simulink model "SIL_Arduino"  (R2022b)
settings: Solver=ode3  StartTime=0.0  StopTime=10.0  FixedStep=0.01  RelTol=1e-3
values from neighbouring files (symbols this model uses):
  Acceleration_Max = 3.2    [Matlab_WorkSpace.mat]
  Distance_initial = 8    [Matlab_WorkSpace.mat]
  Frein_Max = -9    [Matlab_WorkSpace.mat]
  glissement = 0.22    [Matlab_WorkSpace.mat]
  r = 0.3    [Matlab_WorkSpace.mat]
  vehicule_half_length = 2.5    [Matlab_WorkSpace.mat]
libraries: sim3dautolib x2, sim3dprobsensorlib x1, sim3dlib x1, pil_lib x1, slpidlib x1
settings Model: Creator=Yoamiri  LastModifiedBy=Yoamiri
settings OptimizationCC: DefaultParameterBehavior=Inlined  EnhancedBackFolding=on  PassReuseOutputArgsAs=Individual arguments  ZeroExternalMemoryAtStartup=off  ZeroInternalMemoryAtStartup=off  OptimizeBlockOrder=speed  DifferentSizesBufferReuse=on  OptimizationCustomize=off  EfficientTunableParamExpr=on
settings DebuggingCC: ParameterPrecisionLossMsg=none  ParameterTunabilityLossMsg=error
settings HardwareCC: ProdBitPerPointer=32  ProdBitPerSizeT=32  ProdBitPerPtrDiffT=32  ProdLargestAtomicFloat=None  ProdWordSize=32  ProdHWDeviceType=Atmel->AVR (32-bit)
settings SFSimCC: MATLABDynamicMemAlloc=off
settings RTWCC: Description=Embedded Coder  SystemTargetFile=ert.tlc  TemplateMakefile=ert_default_tmf  CreateSILPILBlock=SIL
settings CodeAppCC: ForceParamTrailComments=on  IgnoreCustomStorageClasses=off  OperatorAnnotations=on  SimulinkDataObjDesc=on  SFDataObjDesc=on  InsertBlockDesc=on
settings ERTTargetCC: TargetLangStandard=C99 (ISO)  GenerateSampleERTMain=on  SupportContinuousTime=on  SupportVariableSizeSignals=on  InlinedParameterPlacement=NonHierarchical  ERTCustomFileTemplate=example_file_process.tlc

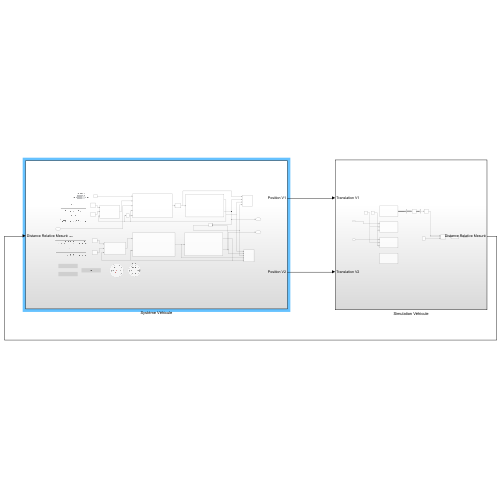
[thumbnail: Simulink's stored preview of the top-level diagram]
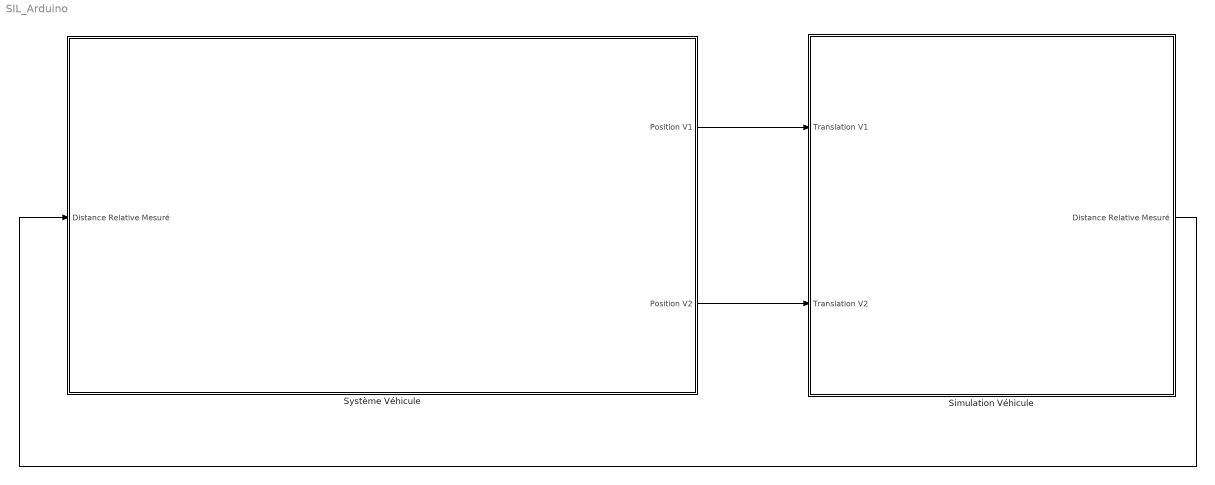
== system SIL_Arduino ==
  Simulation Véhicule : Subsystem
  Système Véhicule : Subsystem
  wires:
  Simulation Véhicule/1(Distance Relative Mesuré) -> Système Véhicule/1(Distance Relative Mesuré)
  Système Véhicule/2(Position V2) -> Simulation Véhicule/2(Translation V2)
  Système Véhicule/1(Position V1) -> Simulation Véhicule/1(Translation V1)

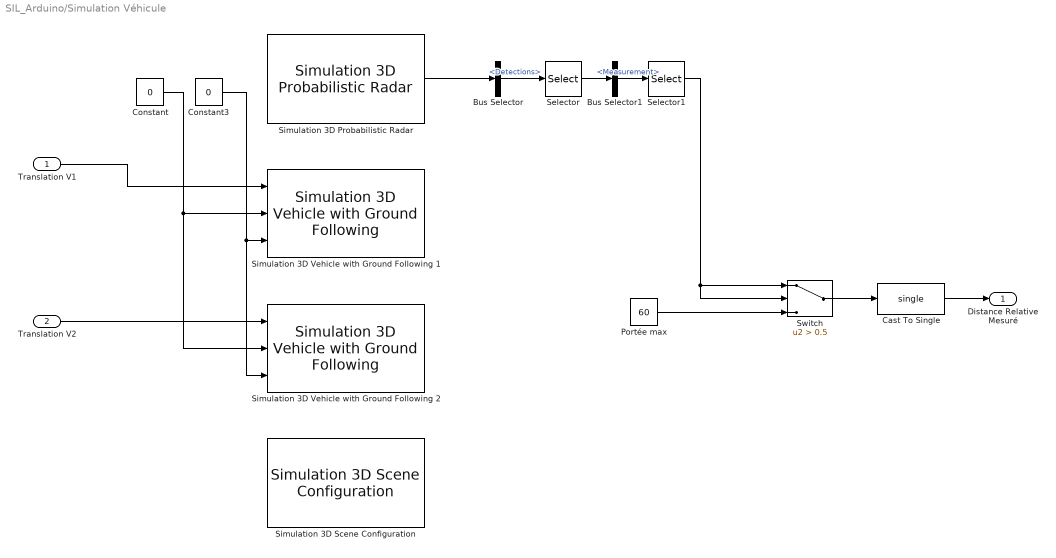
== system SIL_Arduino/Simulation Véhicule ==
  Translation V1 : Inport
  Translation V2 : Inport  Port=2
  Bus Selector : BusSelector  OutputSignals=Detections
  Bus Selector1 : BusSelector  OutputSignals=Measurement
  Cast To Single : DataTypeConversion  OutDataTypeStr=single  SaturateOnIntegerOverflow=off  RndMeth=Floor
  Constant : Constant  Value=0
  Constant3 : Constant  Value=0
  Portée max : Constant  Value=60
  Selector : Selector  InputPortWidth=50  IndexOptions=Index vector (dialog)  Indices=[1]  OutputSizes=1
  Selector1 : Selector  InputPortWidth=6  IndexOptions=Index vector (dialog)  Indices=[1]  OutputSizes=1
  Simulation 3D Probabilistic Radar : sim3dprobsensorlib/Simulation 3D Probabilistic Radar  Priority=1  sensorTag=Sim3dSensor2  sensorId=2  sensorName=Sim3dSensor2  vehTagList={'Scene Origin';'SimulinkVehicle1';'SimulinkVehicle2'}  vehTag=SimulinkVehicle1  mountLoc=Origin  offsetFlag=off  tmountOffset=[2.42, 0, 0.6]  rmountOffset=[0, 0, 0]  AzimuthResolution=4  ElevationResolution=10  RangeResolution=2.5  RangeRateResolution=0.5  AzimuthBiasFraction=0.1  ElevationBiasFraction=0.1  RangeBiasFraction=0.05  RangeRateBiasFraction=0.05  FieldOfView=[ 50, 10 ]  DetectionRange=[ 0.5, 200 ]  RangeRateLimits=[ -100, 100 ]  DetectionProbability=0.95  FalseAlarmRate=1e-6  ReferenceRange=180  ReferenceRCS=-10  HasElevation=on  HasRangeRate=on  HasNoise=on  HasFalseAlarms=on  InitialSeedSource=Repeatable  InitialSeed=0  MaxNumDetections=50  DetectionCoordinates=Ego Cartesian  SpecifyOutputBusName=off  BusName=BusSimulation3DRadarTruthSensor  SampleTime=-1  mountPoint=[0 0 0]  mountOrientation=[0 0 0]  aMode=3  ID=2
      settings: LibrarySourceBlock=drivingsim3d/Simulation 3D Probabilistic Radar
  Simulation 3D Scene Configuration : sim3dlib/Simulation 3D Scene Configuration  Priority=0  ProjectFormat=Default Scenes  SceneDesc=Straight road  ProjectName=C:\Program Files\MATLAB\R2022b\toolbox\shared\sim3d_projects\automotive_project\UE4\WindowsNoEditor\VehicleSimulation.exe  ScenePath=/Game/Maps/HwStrght  EnableOpenDRIVE=off  vehTagList={'Scene Origin';'SimulinkVehicle1';'SimulinkVehicle2'}  vehTag=SimulinkVehicle1  OpVisEn=off  Ts=1/20  EnableWindow=on  EnableRemoteAccess=off  EnableWeather=off  SunAltitude=40.0  SunAzimuth=90  clouds=10  wind=1  fog=0  rain=0  EnableGeospatial=off  OriginHeight=200  OriginLatitude=40.744652  OriginLongitude=-73.988864  MapStyle=Aerial  AdditionalAssetIDs=[]  UseAdvancedSunSky=off  SolarTime=11  TimeZone=-5  Day=21  Month=9  Year=2022  UseDaylightSavingTime=on  DSTStartDay=10  DSTStartMonth=3  DSTEndDay=3  DSTEndMonth=11  DSTSwitchHour=2  sensorTag=MainCamera2  sensorId=2  sensorName=MainCamera2  mountLoc=Origin  offsetFlag=off  tmountOffset=[0, 0, 0]  rmountOffset=[0, 0, 0]  HorizontalResolution=1280  VerticalResolution=720  HorizontalFOV=60  mountPoint=[0 0 0]  mountOrientation=[0 0 0]  aMode=3  ID=2  GeoTrigger=Inactive
      settings: LibrarySourceBlock=drivingsim3d/Simulation 3D Scene Configuration
  Simulation 3D Vehicle with Ground Following 1 : sim3dautolib/Simulation 3D Vehicle with Ground Following  Priority=-1  PassVehMesh=Sedan  MeshPath=/MathWorksAutomotiveContent/Vehicles/Muscle/Meshes/SK_MuscleCar.SK_MuscleCar  TrackWidth=1.9  WheelBase=3  WheelRadius=0.35  VehColor=Blue  InitialPos=[0, 0, 0]  InitialRot=[0, 0, 0]  ActorName=SimulinkVehicle3  SampleTime=-1  ActorType=SimulinkVehicle  ID=3  aMode=3  ActorTag=SimulinkVehicle3  CoordinateScheme=ISO  VehLightsControl=off  HeadlightColor=[ 1, 1, 1 ]  HighBeamIntensity=100000  LowBeamIntensity=60000  HighBeamConeAngle=70  LowBeamConeAngle=70  LeftHeadlightOrientation=[ 0, 0 ]  RightHeadlightOrientation=[ 0, 0 ]  BrakelightIntensity=500  ReverselightIntensity=500  SignallightIntensity=500  SignallightPeriod=1  SignalPulseWidth=50  TransformOutportEnabled=off
      settings: LibrarySourceBlock=drivingsim3d/Simulation 3D Vehicle with Ground Following
  Simulation 3D Vehicle with Ground Following 2 : sim3dautolib/Simulation 3D Vehicle with Ground Following  Priority=-1  PassVehMesh=Sedan  MeshPath=/MathWorksAutomotiveContent/Vehicles/Muscle/Meshes/SK_MuscleCar.SK_MuscleCar  TrackWidth=1.9  WheelBase=3  WheelRadius=0.35  VehColor=White  InitialPos=[0, 0, 0]  InitialRot=[0, 0, 0]  ActorName=SimulinkVehicle4  SampleTime=-1  ActorType=SimulinkVehicle  ID=4  aMode=3  ActorTag=SimulinkVehicle4  CoordinateScheme=ISO  VehLightsControl=off  HeadlightColor=[ 1, 1, 1 ]  HighBeamIntensity=100000  LowBeamIntensity=60000  HighBeamConeAngle=70  LowBeamConeAngle=70  LeftHeadlightOrientation=[ 0, 0 ]  RightHeadlightOrientation=[ 0, 0 ]  BrakelightIntensity=500  ReverselightIntensity=500  SignallightIntensity=500  SignallightPeriod=1  SignalPulseWidth=50  TransformOutportEnabled=off
      settings: LibrarySourceBlock=drivingsim3d/Simulation 3D Vehicle with Ground Following
  Switch : Switch  Criteria=u2 > Threshold  Threshold=0.5  SaturateOnIntegerOverflow=off  InputSameDT=off
  Distance Relative Mesuré : Outport
  wires:
  Constant/1 -> Simulation 3D Vehicle with Ground Following 1/2, Simulation 3D Vehicle with Ground Following 2/2
  Constant3/1 -> Simulation 3D Vehicle with Ground Following 2/3, Simulation 3D Vehicle with Ground Following 1/3
  Simulation 3D Probabilistic Radar/1 -> Bus Selector/1
  Bus Selector/1 -> Selector/1  "<Detections>"
  Selector/1 -> Bus Selector1/1
  Bus Selector1/1 -> Selector1/1  "<Measurement>"
  Translation V2/1 -> Simulation 3D Vehicle with Ground Following 2/1
  Translation V1/1 -> Simulation 3D Vehicle with Ground Following 1/1
  Switch/1 -> Cast To Single/1
  Selector1/1 -> Switch/1, Switch/2
  Portée max/1 -> Switch/3
  Cast To Single/1 -> Distance Relative Mesuré/1

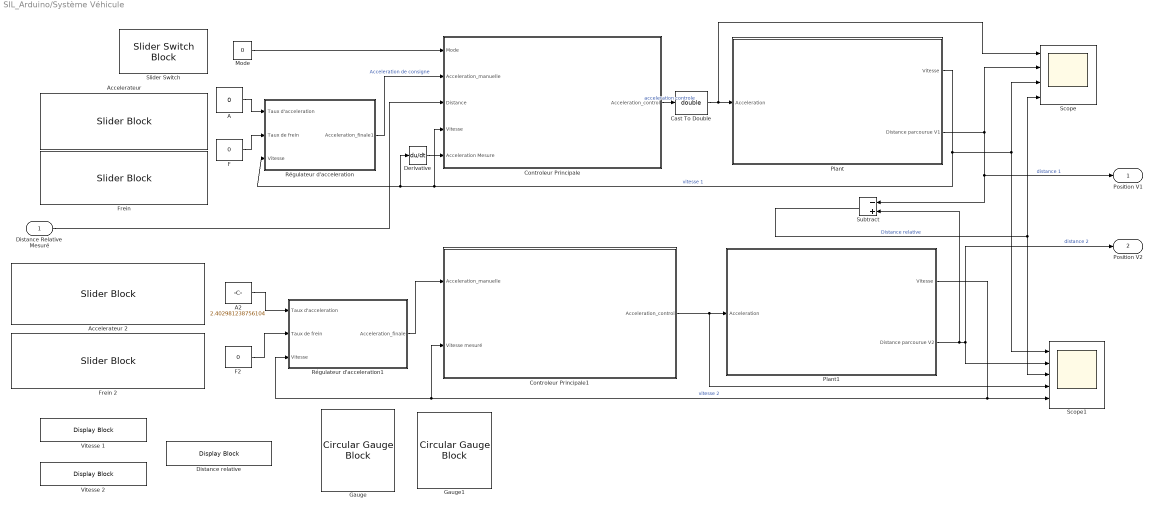
== system SIL_Arduino/Système Véhicule ==
  Distance Relative Mesuré : Inport
  A : Constant  Value=0
  A2 : Constant  Value=2.402981238756104
  Accelerateur : SliderBlock
  Accelerateur 2 : SliderBlock  TickInterval=10
  Cast To Double : DataTypeConversion  OutDataTypeStr=double  SaturateOnIntegerOverflow=off  RndMeth=Floor
  Controleur Principale : Subsystem  DialogController=pil_create_dialog  LoadFcn=|
      | try
      |    if ~strcmp(rtw.pil.getPILVersion, '9.13 (R2022b)_15')
      |       set_param(gcb, 'DialogController', '');
      |       set_param(gcb, 'DialogControllerArgs', '');
      |    end
      | catch e
      |       set_param(gcb, 'DialogController', '');
      |       set_param(gcb, 'DialogControllerArgs', '');
      | end
      mask help: PIL:pil:XILBlockMaskDesc
      mask Display: disp('SIL');
  Controleur Principale1 : Subsystem
  Derivative : Derivative
  Distance relative : DisplayBlock  LabelPosition=Hide  Transparency=1
  F : Constant  Value=0
  F2 : Constant  Value=0
  Frein : SliderBlock
  Frein 2 : SliderBlock  TickInterval=10
  Gauge : CircularGaugeBlock
  Gauge1 : CircularGaugeBlock
  Mode : Constant  Value=0  OutDataTypeStr=boolean
  Plant : Subsystem
  Plant1 : Subsystem
  Régulateur d'acceleration : Subsystem
  Régulateur d'acceleration1 : Subsystem
  Scope : Scope  NumInputPorts=4
  Scope1 : Scope  NumInputPorts=5
  Slider Switch : SliderSwitchBlock
      settings: Values={{'Off', 'On'}, [1 0]}
  Subtract : Sum  Inputs=-+
  Vitesse 1 : DisplayBlock  LabelPosition=Hide  Transparency=1
  Vitesse 2 : DisplayBlock  LabelPosition=Hide  Transparency=1
  Position V1 : Outport
  Position V2 : Outport  Port=2
  wires:
  Controleur Principale1/1(Acceleration_control) -> Plant1/1(Acceleration), Scope1/4
  A2/1 -> Régulateur d'acceleration1/1(Taux d'acceleration)
  Régulateur d'acceleration1/1(Acceleration_finale) -> Controleur Principale1/1(Acceleration_manuelle)
  Régulateur d'acceleration/1(Acceleration_finale1) -> Controleur Principale/2(Acceleration_manuelle)  "Acceleration de consigne"
  Controleur Principale/1(Acceleration_control) -> Cast To Double/1  "acceleration controle"
  F2/1 -> Régulateur d'acceleration1/2(Taux de frein)
  Plant/1(Vitesse) -> Scope/3, Scope1/1, Controleur Principale/4(Vitesse), Derivative/1, Régulateur d'acceleration/3(Vitesse)  "vitesse 1"
  Mode/1 -> Controleur Principale/1(Mode)
  Subtract/1 -> Scope/4, Scope1/3  "Distance relative"
  Plant1/1(Vitesse) -> Régulateur d'acceleration1/3(Vitesse), Controleur Principale1/2(Vitesse mesuré), Scope1/5  "vitesse 2"
  Plant/2(Distance parcourue V1) -> Scope/2, Position V1/1, Subtract/1  "distance 1"
  Plant1/2(Distance parcourue V2) -> Scope1/2, Position V2/1, Subtract/2  "distance 2"
  A/1 -> Régulateur d'acceleration/1(Taux d'acceleration)
  F/1 -> Régulateur d'acceleration/2(Taux de frein)
  Distance Relative Mesuré/1 -> Controleur Principale/3(Distance)
  Cast To Double/1 -> Scope/1, Plant/1(Acceleration)
  Derivative/1 -> Controleur Principale/5(Acceleration Mesure)

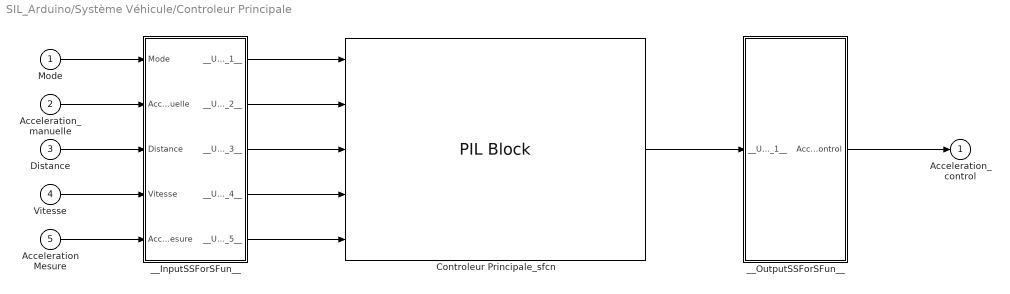
== system SIL_Arduino/Système Véhicule/Controleur Principale ==
  Mode : Inport
  Acceleration_manuelle : Inport  Port=2
  Distance : Inport  Port=3
  Vitesse : Inport  Port=4
  Acceleration Mesure : Inport  Port=5
  Controleur Principale_sfcn : pil_lib/PIL Block  SimulationMode=SIL  IsTopModelPIL=off  CodeDir=Controleur_ert_rtw  AnchorDir=C:\Users\Yoamiri\Desktop\Projet-Controle d'espacement en file de vehicules\MIL-Principale Modèle  ConfigName=Software-in-the-Loop (SIL)  XrelIsTopModelCode=on  XrelIsReusable=off  XrelDWorkNames={}  XrelDWorkTypes={}  XrelModelArgVals={}  XrelOrderedParamNames={}
  __InputSSForSFun__ : Subsystem
  __OutputSSForSFun__ : Subsystem
  Acceleration_control : Outport
  wires:
  Mode/1 -> __InputSSForSFun__/1(Mode)
  Acceleration_manuelle/1 -> __InputSSForSFun__/2(Acceleration_manuelle)
  Distance/1 -> __InputSSForSFun__/3(Distance)
  Vitesse/1 -> __InputSSForSFun__/4(Vitesse)
  Acceleration Mesure/1 -> __InputSSForSFun__/5(Acceleration Mesure)
  __InputSSForSFun__/1(__UniqueOutportName__1__) -> Controleur Principale_sfcn/1
  __InputSSForSFun__/2(__UniqueOutportName__2__) -> Controleur Principale_sfcn/2
  __InputSSForSFun__/3(__UniqueOutportName__3__) -> Controleur Principale_sfcn/3
  __InputSSForSFun__/4(__UniqueOutportName__4__) -> Controleur Principale_sfcn/4
  __InputSSForSFun__/5(__UniqueOutportName__5__) -> Controleur Principale_sfcn/5
  Controleur Principale_sfcn/1 -> __OutputSSForSFun__/1(__UniqueInportName__1__)
  __OutputSSForSFun__/1(Acceleration_control) -> Acceleration_control/1

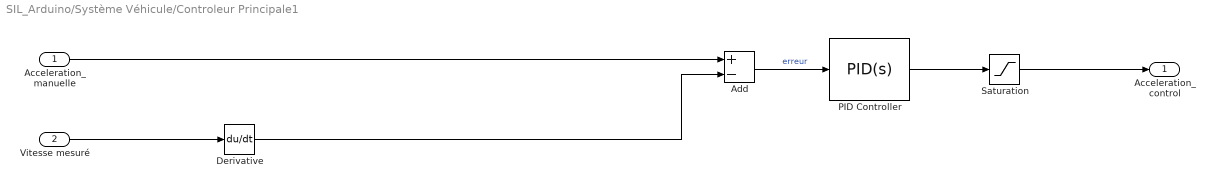
== system SIL_Arduino/Système Véhicule/Controleur Principale1 ==
  Acceleration_manuelle : Inport
  Vitesse mesuré : Inport  Port=2
  Add : Sum  Inputs=+-
  Derivative : Derivative
  PID Controller : slpidlib/PID Controller  Controller=PID  Form=Parallel  TimeDomain=Continuous-time  UseExternalTs=off  SampleTime=-1  IntegratorMethod=Forward Euler  FilterMethod=Forward Euler  ControllerParametersSource=internal  P=4  I=1.5  UseKiTs=off  D=0  N=100  UseFilter=on  TunerSelectOption=Transfer Function Based (PID Tuner App)  InitialConditionSource=internal  InitialConditionForIntegrator=0  InitialConditionForFilter=0  DifferentiatorICPrevScaledInput=0  ExternalReset=none  TrackingMode=off  Kt=1  LimitOutput=off  SatLimitsSource=internal  UpperSaturationLimit=inf  LowerSaturationLimit=-inf  LinearizeAsGain=on  AntiWindupMode=none  Kb=1  LimitIntegrator=off  UpperIntegratorSaturationLimit=inf  LowerIntegratorSaturationLimit=-inf  POutMin=[]  POutMax=[]  IOutMin=[]  IOutMax=[]  DOutMin=[]  DOutMax=[]  NOutMin=[]  NOutMax=[]  SumOutMin=[]  SumOutMax=[]  SaturationOutMin=[]  SaturationOutMax=[]  PParamMin=[]  PParamMax=[]  IParamMin=[]  IParamMax=[]  DParamMin=[]  DParamMax=[]  NParamMin=[]  NParamMax=[]  KbParamMin=[]  KbParamMax=[]  KtParamMin=[]  KtParamMax=[]  KbOutMin=[]  KbOutMax=[]  KtOutMin=[]  KtOutMax=[]  IntegratorOutMin=[]  IntegratorOutMax=[]  FilterOutMin=[]  FilterOutMax=[]  SumI1OutMin=[]  SumI1OutMax=[]  SumI2OutMin=[]  SumI2OutMax=[]  SumI3OutMin=[]  SumI3OutMax=[]  SumI4OutMin=[]  SumI4OutMax=[]  SumDOutMin=[]  SumDOutMax=[]  DifferentiatorOutMin=[]  DifferentiatorOutMax=[]  FilterDiffOutCoefMin=[]  FilterDiffOutCoefMax=[]  ReciprocalOutMin=[]  ReciprocalOutMax=[]  SumDenOutMin=[]  SumDenOutMax=[]  SumNumOutMin=[]  SumNumOutMax=[]  DivideOutMin=[]  DivideOutMax=[]  UdiffTsProdOutMin=[]  UdiffTsProdOutMax=[]  NTsProdOutMin=[]  NTsProdOutMax=[]  UintegralTsProdOutMin=[]  UintegralTsProdOutMax=[]  UngainTsProdOutMin=[]  UngainTsProdOutMax=[]  ClampingZeroOutDataTypeStr=Inherit: Inherit via back propagation  ClampingZeroOutMin=[]  ClampingZeroOutMax=[]  FilterDenConstantOutDataTypeStr=Inherit: Inherit via back propagation  FilterDenConstantOutMin=[]  FilterDenConstantOutMax=[]  PCopyOutDataTypeStr=Inherit: Inherit via back propagation  PCopyOutMin=[]  PCopyOutMax=[]  NCopyOutDataTypeStr=Inherit: Inherit via back propagation  NCopyOutMin=[]  NCopyOutMax=[]  IntegratorContinuousStateAttributes=''  IntegratorStateMustResolveToSignalObject=off  IntegratorRTWStateStorageClass=Auto  FilterContinuousStateAttributes=''  FilterStateMustResolveToSignalObject=off  FilterRTWStateStorageClass=Auto  ParallelPVariant=InternalParameters  IdealPVariant=Disabled  IVariant=InternalParameters  DVariant=InternalParameters  IntegratorVariant=Continuous  SatVariant=Disabled  AWVariant=Passthrough  PCopyVariant=Disabled  TRVariant=Disabled  FdbkBlocksVariant=Forward  IdealPFdbkVariant=Disabled  SatFdbkVariant=Disabled  DerivativeFilterVariant=ContFilter  NVariant=InternalParameters  NCopyVariant=Disabled  FilterICVariant=InternalICsFilter  IntegratorICVariant=InternalICs  ExternalResetVariant=Disabled  TRSumVariant=Passthrough  SumFdbkVariant=Disabled  SumVariant=Sum_PID  TsampFilterVariant=InternalTs  TsampNgainVariant=Passthrough  TsampIntegralVariant=Passthrough  ExternalSaturationOutDataTypeStr=Inherit: Same as second input
  Saturation : Saturate  UpperLimit=Acceleration_Max  LowerLimit=Frein_Max
  Acceleration_control : Outport
  wires:
  Vitesse mesuré/1 -> Derivative/1
  Derivative/1 -> Add/2
  Add/1 -> PID Controller/1  "erreur"
  PID Controller/1 -> Saturation/1
  Acceleration_manuelle/1 -> Add/1
  Saturation/1 -> Acceleration_control/1

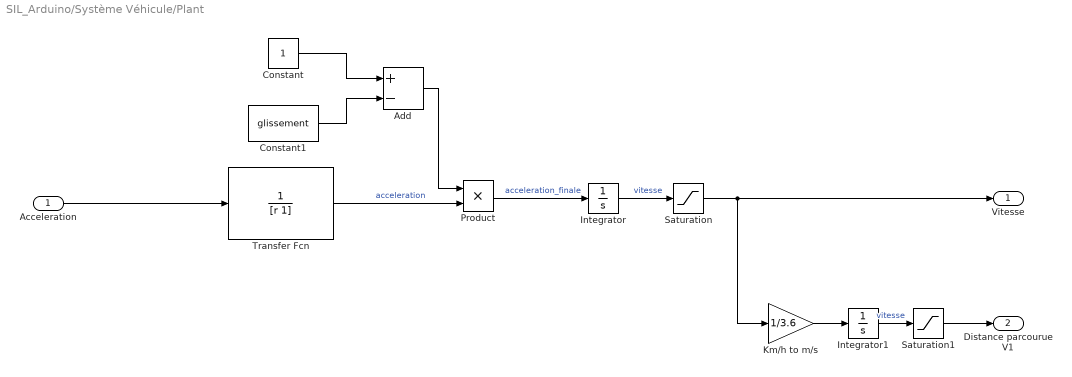
== system SIL_Arduino/Système Véhicule/Plant ==
  Acceleration : Inport
  Add : Sum  Inputs=+-
  Constant : Constant
  Constant1 : Constant  Value=glissement
  Integrator : Integrator
  Integrator1 : Integrator
  Km/h to m/s : Gain  Gain=1/3.6
  Product : Product
  Saturation : Saturate  UpperLimit=120  LowerLimit=0
  Saturation1 : Saturate  UpperLimit=inf  LowerLimit=0
  Transfer Fcn : TransferFcn  Denominator=[r 1]
  Vitesse : Outport
  Distance parcourue V1 : Outport  Port=2
  wires:
  Acceleration/1 -> Transfer Fcn/1
  Product/1 -> Integrator/1  "acceleration_finale"
  Transfer Fcn/1 -> Product/2  "acceleration"
  Constant/1 -> Add/1
  Constant1/1 -> Add/2
  Add/1 -> Product/1
  Integrator1/1 -> Saturation1/1  "vitesse"
  Saturation/1 -> Vitesse/1, Km/h to m/s/1
  Saturation1/1 -> Distance parcourue V1/1
  Km/h to m/s/1 -> Integrator1/1
  Integrator/1 -> Saturation/1  "vitesse"

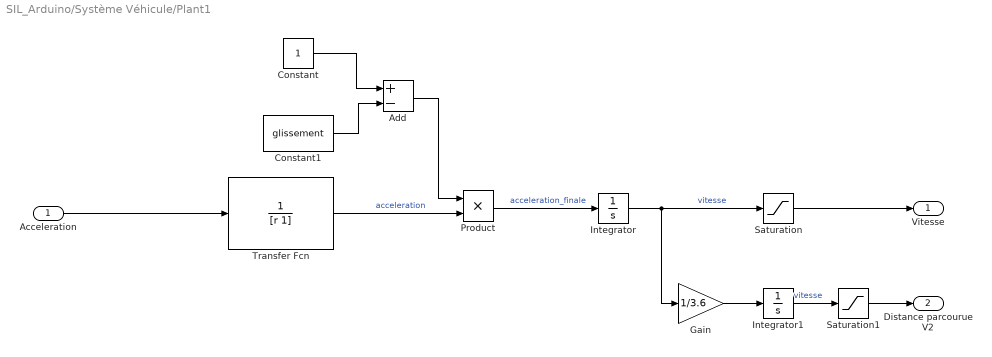
== system SIL_Arduino/Système Véhicule/Plant1 ==
  Acceleration : Inport
  Add : Sum  Inputs=+-
  Constant : Constant
  Constant1 : Constant  Value=glissement
  Gain : Gain  Gain=1/3.6
  Integrator : Integrator
  Integrator1 : Integrator  InitialCondition=Distance_initial+vehicule_half_length
  Product : Product
  Saturation : Saturate  UpperLimit=120  LowerLimit=0
  Saturation1 : Saturate  UpperLimit=inf  LowerLimit=0
  Transfer Fcn : TransferFcn  Denominator=[r 1]
  Vitesse : Outport
  Distance parcourue V2 : Outport  Port=2
  wires:
  Acceleration/1 -> Transfer Fcn/1
  Product/1 -> Integrator/1  "acceleration_finale"
  Transfer Fcn/1 -> Product/2  "acceleration"
  Constant/1 -> Add/1
  Constant1/1 -> Add/2
  Add/1 -> Product/1
  Integrator/1 -> Saturation/1, Gain/1  "vitesse"
  Integrator1/1 -> Saturation1/1  "vitesse"
  Gain/1 -> Integrator1/1
  Saturation/1 -> Vitesse/1
  Saturation1/1 -> Distance parcourue V2/1

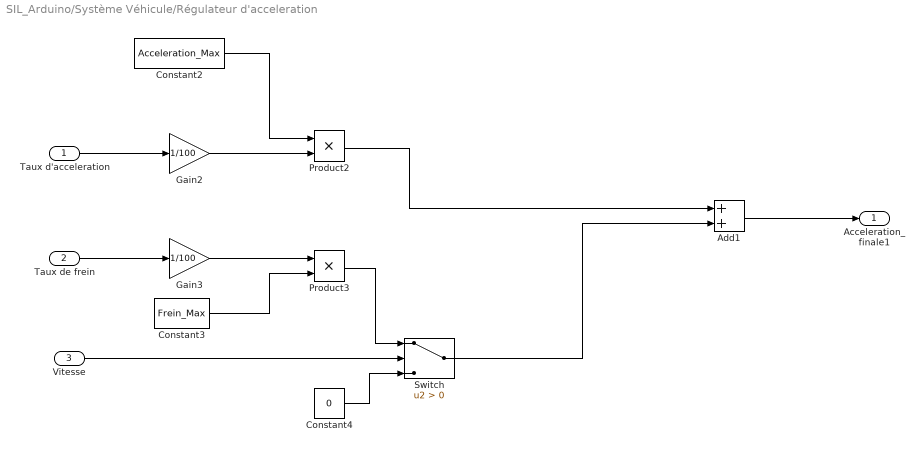
== system SIL_Arduino/Système Véhicule/Régulateur d'acceleration ==
  Taux d'acceleration : Inport
  Taux de frein : Inport  Port=2
  Vitesse : Inport  Port=3
  Add1 : Sum
  Constant2 : Constant  Value=Acceleration_Max
  Constant3 : Constant  Value=Frein_Max
  Constant4 : Constant  Value=0
  Gain2 : Gain  Gain=1/100
  Gain3 : Gain  Gain=1/100
  Product2 : Product
  Product3 : Product
  Switch : Switch  Criteria=u2 > Threshold  SaturateOnIntegerOverflow=off  InputSameDT=off
  Acceleration_finale1 : Outport
  wires:
  Constant4/1 -> Switch/3
  Product3/1 -> Switch/1
  Vitesse/1 -> Switch/2
  Switch/1 -> Add1/2
  Product2/1 -> Add1/1
  Taux d'acceleration/1 -> Gain2/1
  Gain3/1 -> Product3/1
  Add1/1 -> Acceleration_finale1/1
  Constant2/1 -> Product2/1
  Taux de frein/1 -> Gain3/1
  Gain2/1 -> Product2/2
  Constant3/1 -> Product3/2

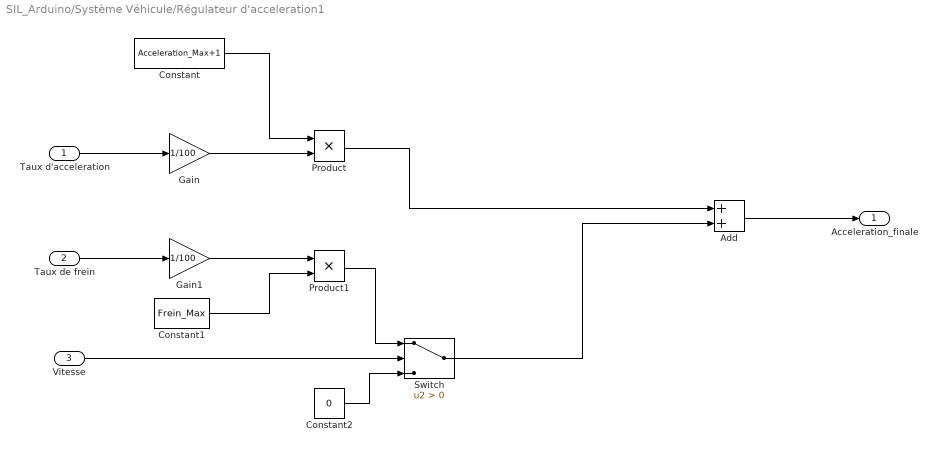
== system SIL_Arduino/Système Véhicule/Régulateur d'acceleration1 ==
  Taux d'acceleration : Inport
  Taux de frein : Inport  Port=2
  Vitesse : Inport  Port=3
  Add : Sum
  Constant : Constant  Value=Acceleration_Max+1
  Constant1 : Constant  Value=Frein_Max
  Constant2 : Constant  Value=0
  Gain : Gain  Gain=1/100
  Gain1 : Gain  Gain=1/100
  Product : Product
  Product1 : Product
  Switch : Switch  Criteria=u2 > Threshold  SaturateOnIntegerOverflow=off  InputSameDT=off
  Acceleration_finale : Outport
  wires:
  Taux de frein/1 -> Gain1/1
  Taux d'acceleration/1 -> Gain/1
  Constant1/1 -> Product1/2
  Constant/1 -> Product/1
  Gain/1 -> Product/2
  Gain1/1 -> Product1/1
  Product/1 -> Add/1
  Add/1 -> Acceleration_finale/1
  Vitesse/1 -> Switch/2
  Product1/1 -> Switch/1
  Switch/1 -> Add/2
  Constant2/1 -> Switch/3

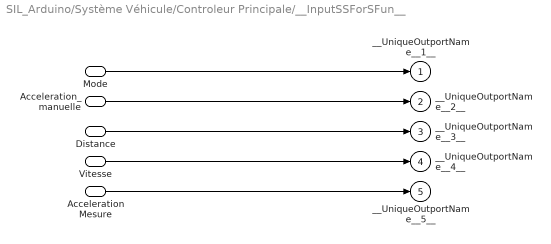
== system SIL_Arduino/Système Véhicule/Controleur Principale/__InputSSForSFun__ ==
  Mode : Inport
  Acceleration_manuelle : Inport  Port=2
  Distance : Inport  Port=3
  Vitesse : Inport  Port=4
  Acceleration Mesure : Inport  Port=5
  __UniqueOutportName__1__ : Outport
  __UniqueOutportName__2__ : Outport  Port=2
  __UniqueOutportName__3__ : Outport  Port=3
  __UniqueOutportName__4__ : Outport  Port=4
  __UniqueOutportName__5__ : Outport  Port=5
  wires:
  Mode/1 -> __UniqueOutportName__1__/1
  Acceleration_manuelle/1 -> __UniqueOutportName__2__/1
  Distance/1 -> __UniqueOutportName__3__/1
  Vitesse/1 -> __UniqueOutportName__4__/1
  Acceleration Mesure/1 -> __UniqueOutportName__5__/1

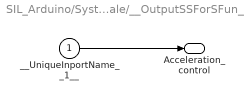
== system SIL_Arduino/Système Véhicule/Controleur Principale/__OutputSSForSFun__ ==
  __UniqueInportName__1__ : Inport
  Acceleration_control : Outport
  wires:
  __UniqueInportName__1__/1 -> Acceleration_control/1
